simulink model "prob5"  (R2020a)
settings: Solver=VariableStepAuto  StartTime=0.0  StopTime=10.0  RelTol=1e-3
values from neighbouring files (symbols this model uses):
  C = 9.9999999999999991E-6    [data.sldd]    (also in para.m = 1e-05)
  R = 10.0    [data.sldd]    (also in para.m = 10)
  V = 1.0    [data.sldd]    (also in para.m = 5)
settings Model: Creator=vijay  LastModifiedBy=vijay

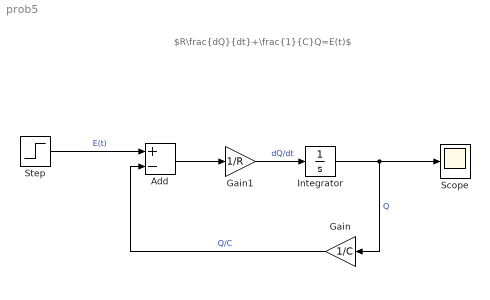
== system prob5 ==
  note: $R\frac{dQ}{dt}+\frac{1}{C}Q=E(t)$
  Add : Sum  Inputs=+-
  Gain : Gain  Gain=1/C
  Gain1 : Gain  Gain=1/R
  Integrator : Integrator
  Scope : Scope
  Step : Step  Time=V  SampleTime=0
  wires:
  Step/1 -> Add/1  "E(t)"
  Integrator/1 -> Gain/1, Scope/1  "Q"
  Gain1/1 -> Integrator/1  "dQ/dt"
  Add/1 -> Gain1/1
  Gain/1 -> Add/2  "Q/C"
